simulink model "control_nolineal_entrada_estado"  (R2018a)
settings: Solver=VariableStepAuto  StartTime=0.0  StopTime=10.0  RelTol=1e-3
InitFcn:
  | control_nolineal_linealizacion_entrada_estado
values from neighbouring files (symbols this model uses):
  ki = kt(1,3)    [control_nolineal_linealizacion_entrada_estado.m]    (also in e_mimo.m; ej_mimo.m = kt(:,2+1:end); ej_mimo2.m = kt(:,2+1:end); ejemplo_2.m)
  kii = kt(1,3)    [control_nolineal_linealizacion_entrada_estado.m]    (also in control_nolineal_linealizacion_entrada_estado2.m)
  kp = kt(1,1:2)    [control_nolineal_linealizacion_entrada_estado.m]    (also in e_mimo.m; ej_mimo.m = kt(:,1:2); ej_mimo2.m = kt(:,1:2); ejemplo_2.m)
  kpi = kt(1,1:2)    [control_nolineal_linealizacion_entrada_estado.m]    (also in control_nolineal_linealizacion_entrada_estado2.m)
libraries: simulink x2
settings Model: Creator=carma  LastModifiedBy=carma

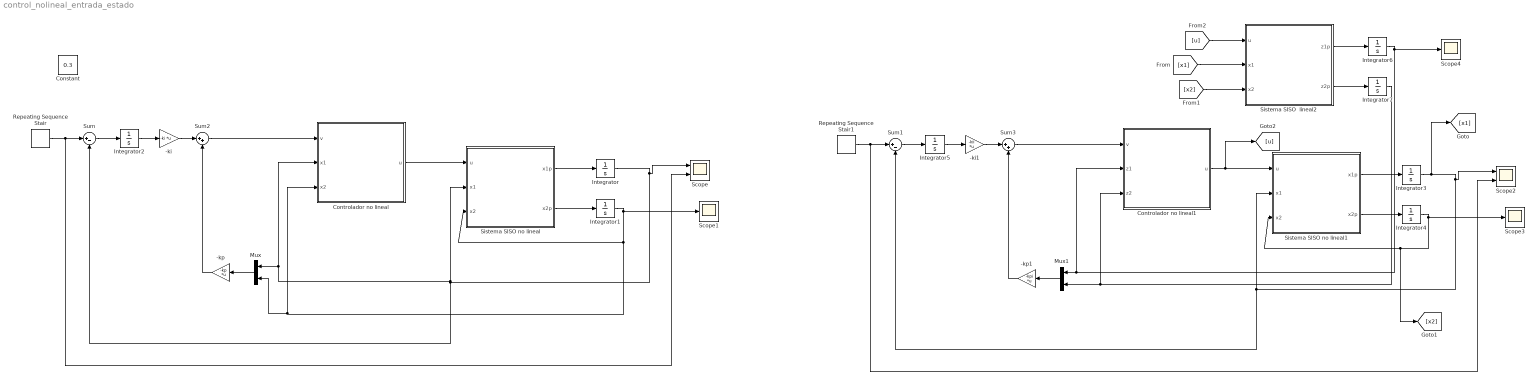
== system control_nolineal_entrada_estado ==
  -ki : Gain  Gain=-ki  Multiplication=Matrix(K*u) (u vector)
  -ki1 : Gain  Gain=-kii  Multiplication=Matrix(K*u) (u vector)
  -kp : Gain  Gain=-kp  Multiplication=Matrix(K*u) (u vector)
  -kp1 : Gain  Gain=-kpi  Multiplication=Matrix(K*u) (u vector)
  Constant : Constant  Value=0.3
  Controlador no lineal : MATLAB Function  TreatAsAtomicUnit=on
  Controlador no lineal1 : MATLAB Function  TreatAsAtomicUnit=on
  Integrator{,1..7} (8 alike) : Integrator
  Mux : Mux  Inputs=2
  Mux1 : Mux  Inputs=2
  Repeating Sequence Stair : simulink/Sources/Repeating Sequence Stair  OutValues=[0.5 0.4 -0.2 0.1 0.3].'  tsamp=1  OutMin=[]  OutMax=[]  OutDataTypeStr=double  OutputDataTypeScalingMode=double  OutDataType=fixdt(0,8)  ConRadixGroup=Best Precision: Vector-wise  OutScaling=2^-12
  Repeating Sequence Stair1 : simulink/Sources/Repeating Sequence Stair  OutValues=[0.5 0.4 -0.2 0.1 0.3].'  tsamp=1  OutMin=[]  OutMax=[]  OutDataTypeStr=double  OutputDataTypeScalingMode=double  OutDataType=fixdt(0,8)  ConRadixGroup=Best Precision: Vector-wise  OutScaling=2^-12
  Scope : Scope  NumInputPorts=2
  Scope1 : Scope
  Scope2 : Scope  NumInputPorts=2
  Scope3 : Scope
  Scope4 : Scope
  Sistema SISO  lineal2 : MATLAB Function  TreatAsAtomicUnit=on
  Sistema SISO no lineal : MATLAB Function  TreatAsAtomicUnit=on
  Sistema SISO no lineal1 : MATLAB Function  TreatAsAtomicUnit=on
  Sum : Sum  Inputs=|+-
  Sum1 : Sum  Inputs=|+-
  Sum2 : Sum  Inputs=|++
  Sum3 : Sum  Inputs=|++
  wires:
  Sistema SISO no lineal/1(x1p) -> Integrator/1
  Sistema SISO no lineal/2(x2p) -> Integrator1/1
  Integrator1/1 -> Scope1/1, Mux/2, Controlador no lineal/3(x2), Sistema SISO no lineal/3(x2)
  Controlador no lineal/1(u) -> Sistema SISO no lineal/1(u)
  -ki/1 -> Sum2/1
  Integrator2/1 -> -ki/1
  Sum/1 -> Integrator2/1
  Sum2/1 -> Controlador no lineal/1(v)
  -kp/1 -> Sum2/2
  Mux/1 -> -kp/1
  Integrator/1 -> Scope/1, Sum/2, Mux/1, Controlador no lineal/2(x1), Sistema SISO no lineal/2(x1)
  Repeating Sequence Stair/1 -> Scope/2, Sum/1
  Repeating Sequence Stair1/1 -> Scope2/2, Sum1/1
  Sum3/1 -> Controlador no lineal1/1(v)
  -kp1/1 -> Sum3/2
  Sum1/1 -> Integrator5/1
  Integrator3/1 -> [x1], Scope2/1, Sum1/2, Sistema SISO no lineal1/2(x1)
  Integrator4/1 -> Scope3/1, [x2], Sistema SISO no lineal1/3(x2)
  Integrator5/1 -> -ki1/1
  Sistema SISO no lineal1/1(x1p) -> Integrator3/1
  -ki1/1 -> Sum3/1
  Mux1/1 -> -kp1/1
  Sistema SISO no lineal1/2(x2p) -> Integrator4/1
  Controlador no lineal1/1(u) -> [u], Sistema SISO no lineal1/1(u)
  Sistema SISO  lineal2/1(z1p) -> Integrator6/1
  Sistema SISO  lineal2/2(z2p) -> Integrator7/1
  Integrator6/1 -> Scope4/1, Controlador no lineal1/2(z1), Mux1/1
  Integrator7/1 -> Controlador no lineal1/3(z2), Mux1/2
  [x1] -> Sistema SISO  lineal2/2(x1)
  [x2] -> Sistema SISO  lineal2/3(x2)
  [u] -> Sistema SISO  lineal2/1(u)

== matlab function control_nolineal_entrada_estado/Controlador no lineal ==
  data: v input; u output; x1 input; x2 input
function u = fcn(v,x1,x2)

%parametros
a=4;
c=1;
delta=0.5;

u=(a/c)*(sin(x1+delta)-sin(delta))+v/c;;

%s=5;
%syms y
%Cx3=(2+10^(pk2-y))/(1+10^(pk2-y)+10^(pk1+pk2-2*y));
%h=-x1+x2-x3*Cx3+10^(-y)-10^(y-pkw)==0;

%s=double(solve(h));

== matlab function control_nolineal_entrada_estado/Sistema SISO no lineal ==
  data: u input; x1p output; x1 input; x2 input; x2p output
function [x1p,x2p]= fcn(u,x1,x2)

%parametros
a=4;
b=2;
c=1;
delta=0.5;

x1p=x2;
x2p=-a*(sin(x1+delta)-sin(delta))-b*x2+c*u;

%s=5;
%syms y
%Cx3=(2+10^(pk2-y))/(1+10^(pk2-y)+10^(pk1+pk2-2*y));
%h=-x1+x2-x3*Cx3+10^(-y)-10^(y-pkw)==0;

%s=double(solve(h));

== matlab function control_nolineal_entrada_estado/Controlador no lineal1 ==
  data: v input; u output; z1 input; z2 input
function u = fcn(v,z1,z2)

%parametros
a=4;


u=z1^2+v/(a*cos(asin(z2/a)))

%s=5;
%syms y
%Cx3=(2+10^(pk2-y))/(1+10^(pk2-y)+10^(pk1+pk2-2*y));
%h=-x1+x2-x3*Cx3+10^(-y)-10^(y-pkw)==0;

%s=double(solve(h));

== matlab function control_nolineal_entrada_estado/Sistema SISO no lineal1 ==
  data: u input; x1p output; x1 input; x2 input; x2p output
function [x1p,x2p]= fcn(u,x1,x2)

%parametros
a=4;



x1p=a*sin(x2);
x2p=-x1^2+u;

%s=5;
%syms y
%Cx3=(2+10^(pk2-y))/(1+10^(pk2-y)+10^(pk1+pk2-2*y));
%h=-x1+x2-x3*Cx3+10^(-y)-10^(y-pkw)==0;

%s=double(solve(h));

== matlab function control_nolineal_entrada_estado/Sistema SISO  lineal2 ==
  data: u input; z1p output; x1 input; x2 input; z2p output
function [z1p,z2p]= fcn(u,x1,x2)

%parametros
a=4;


% 
% z1p=z2;
% z2p=v;

z1p=a*sin(x2);
z2p=a*cos(x2)*(-x1^2+u);

%s=5;
%syms y
%Cx3=(2+10^(pk2-y))/(1+10^(pk2-y)+10^(pk1+pk2-2*y));
%h=-x1+x2-x3*Cx3+10^(-y)-10^(y-pkw)==0;

%s=double(solve(h));
